simulink model "ClosedLoop_V1"  (R2021b)
settings: Solver=ode4  StartTime=0.0  StopTime=TMax  FixedStep=DT  MaxStep=DT  RelTol=1e-3  EnableMultiTasking=on
undefined symbols (not defined in the file or in its folder): CertificationSettings, Control, DiscIntNeverNeededParam, Drivetrain, OutList, P_InitAngle, RPM_Init, sigbuilder_block, SimConfig, strmatch
libraries: simulink_extras x4, simulink x1
(part 1 of 3)
settings Model: Creator=bjonkman  LastModifiedBy=LaborAdmin
settings SolverCC: AlgebraicLoopSolver=TrustRegion
settings DataIOCC: LimitDataPoints=on  SaveFormat=Array  SignalLoggingSaveFormat=ModelDataLogs  SaveOutput=off  SaveTime=off  ReturnWorkspaceOutputs=off  SignalLoggingName=sigsOut
settings OptimizationCC: ExpressionDepthLimit=2147483647  LifeSpan=inf
settings DebuggingCC: SaveWithParameterizedLinksMsg=none  UnderspecifiedInitializationDetection=Classic  MergeDetectMultiDrivingBlocksExec=none  SignalResolutionControl=TryResolveAllWithWarning  MultiTaskDSMMsg=warning  MultiTaskCondExecSysMsg=none  FcnCallInpInsideContextMsg=warning  StateNameClashWarn=warning  SFUnexpectedBacktrackingDiag=warning  SFNoUnconditionalDefaultTransitionDiag=warning  SFExecutionAtInitializationDiag=none  SFMachineParentedDataDiag=warning  ArithmeticOperatorsInVariantConditions=warning
settings HardwareCC: ProdBitPerPointer=32  ProdBitPerSizeT=32  ProdBitPerPtrDiffT=32  ProdLargestAtomicFloat=None  ProdIntDivRoundTo=Undefined  ProdEndianess=Unspecified  ProdWordSize=32  ProdHWDeviceType=32-bit Generic  TargetUnknown=on
settings ModelReferenceCC: PropagateSignalLabelsOutOfModel=off
settings SFSimCC: SimUseLocalCustomCode=off  CustomCodeUndefinedFunction=UseInterfaceOnly
settings RTWCC: RTWUseLocalCustomCode=off
settings CodeAppCC: StateflowObjectComments=on
settings GRTTargetCC: TargetLangStandard=C89/C90 (ANSI)  CombineOutputUpdateFcns=off  GRTInterface=on
settings ConfigComp: CovMetricSettings=dw  CovSaveCumulativeToWorkspaceVar=on  CovSaveSingleToWorkspaceVar=on  CovExternalEMLEnable=off

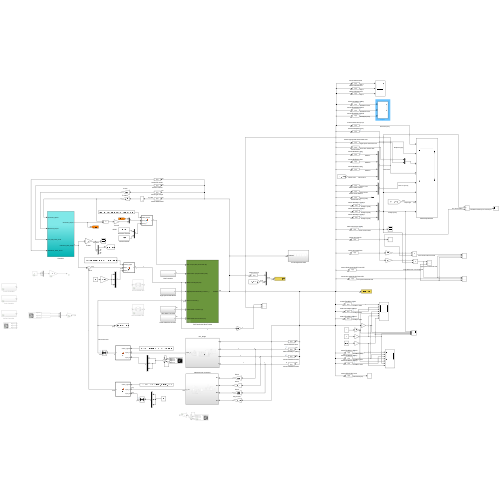
[thumbnail: Simulink's stored preview of the top-level diagram]
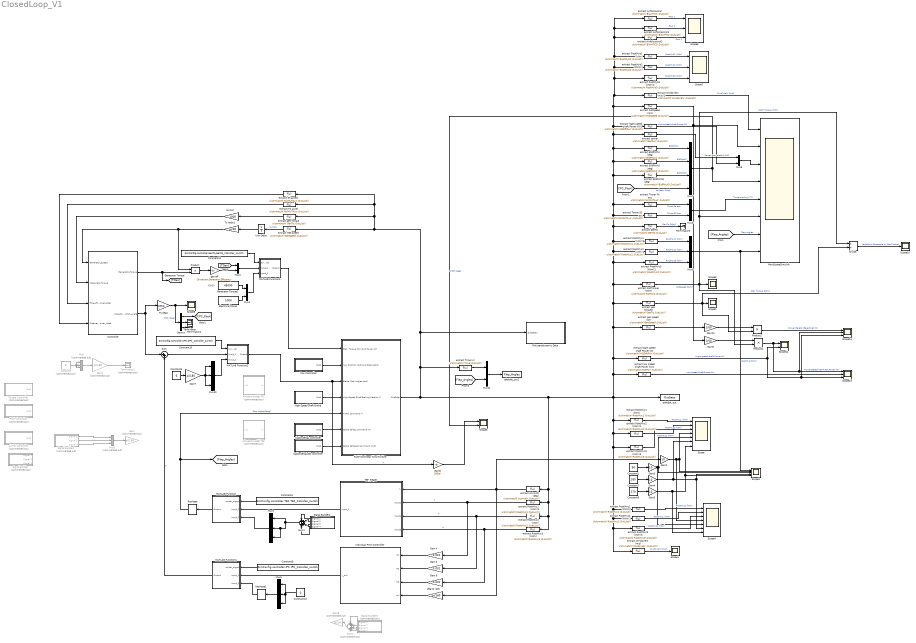
== system ClosedLoop_V1 ==
  note: 43000
  AirFoil Controller : Subsystem  Commented=on
  Aktuatormodell IPC : Subsystem  Commented=on
  Aktuatormodell TEF : Subsystem  Commented=on
  Cable deltaL controller : Subsystem
  Cable deltaLdot controller : Subsystem
  Constant : Constant  Commented=on  Value=6
  Constant1 : Constant  Value=90
  Constant10 : Constant  Value=SimConfig.controller.CPC.CPC_Cotroller_switch
  Constant11 : Constant  Value=SimConfig.controller.GenTq.GenTq_Cotroller_switch
  Constant13 : Constant  Value=0
  Constant3 : Constant  Value=SimConfig.controller.TEF.TEF_Cotroller_switch
  Constant5 : Constant  Value=SimConfig.controller.IPC.IPC_Cotroller_switch
  Constant6 : Constant  Value=6
  Constant7 : Constant  Value=180
  Constant9 : Constant  Value=270
  Controller : Subsystem
  Demux : Demux  Outputs=3
  Divide : Product  Inputs=*/
  Electrical Power : Constant  Value=1000
  FAST Nonlinear Wind Turbine : Subsystem  mask(FAST Nonlinear Wind Turbine){}
      mask help: This block contains the FAST S-Function.
      mask init:
      | clear FAST_SFunc
  Gain : Gain  Commented=on  Gain=pi/180
  Gain 4 : Gain  Gain=0.001
  Gain 5 : Gain  Gain=0.001
  Gain 6 : Gain  Gain=0.001
  Gain1 : Gain  Commented=on  Gain=pi/180
  Gain10 : Gain  Gain=1/60
  Gain{2..5} (4 alike) : Gain  Gain=10
  Gain6 : Gain  Gain=180/pi
  Gain7 : Gain  Gain=pi/180
  Gain8 : Gain  Commented=on  Gain=pi/180
  Gain9 : Gain  Gain=1/60
  Generator Torque2 : Constant  Value=45000
  High-Speed Shaft Brake : Subsystem
  Individual Pitch Controller : Subsystem
  MATLAB Function : MATLAB Function  TreatAsAtomicUnit=on
  MATLAB Function1 : MATLAB Function  TreatAsAtomicUnit=on
  MATLAB Function2 : MATLAB Function  TreatAsAtomicUnit=on
  MATLAB Function3 : MATLAB Function  TreatAsAtomicUnit=on
  MainScopeSimulink : Scope  NumInputPorts=8
  Mux : Mux  Commented=on  Inputs=3
  Mux1 : Mux  Commented=on  Inputs=3
  Mux{3,5,9..10} (4 alike) : Mux  Inputs=3
  Mux{2,4,6,8,11} (5 alike) : Mux  Inputs=2
  Mux7 : Mux
  Pitch Controller : Subsystem  Commented=on
  Plot aerodynamic Data : Subsystem
  Product : Product  RndMeth=Zero
  Product1 : Product
  Product2 : Product
  Reshape : Reshape  OutputDimensionality=Row vector (2-D)  OutputDimensions=[1,3]
  Reshape1 : Reshape  OutputDimensionality=Row vector (2-D)  OutputDimensions=[1,3]
  Scope : Scope  NumInputPorts=7
  Scope{1..2,6,8,15} (5 alike) : Scope
  Scope11 : Scope  NumInputPorts=2
  Scope{7,9,13..14} (4 alike) : Scope  NumInputPorts=3
  Scope3 : Scope  NumInputPorts=5
  Scope4 : Scope  NumInputPorts=7
  Scope5 : Scope  NumInputPorts=2
  Signal Builder : Subsystem  Tag=STV Subsys  Commented=on  LoadFcn=sigbuilder_block('load');  StartFcn=sigbuilder_block('start');  StopFcn=sigbuilder_block('stop');  ClipboardFcn=sigbuilder_block('clipboard');  mask(Sigbuilder block){tuvar=[0:10]}
      mask help: Simulink:masks:SigbuilderBlock_MD
      mask init:
      | if ~strcmp(get_param(bdroot(gcbh),'SimulationStatus'),'stopped') tuvar = sigbuilder_block('maskInit'); end
      settings: CopyFcn=sigbuilder_block('copy');  DeleteFcn=sigbuilder_block('delete');  ModelCloseFcn=sigbuilder_block('modelClose');  PreSaveFcn=sigbuilder_block('preSave');  PauseFcn=sigbuilder_block('pause');  ContinueFcn=sigbuilder_block('continue');  NameChangeFcn=sigbuilder_block('namechange');  OpenFcn=sigbuilder_block('open',[1778.25 246.75 675 420.75 ]);  CloseFcn=sigbuilder_block('close');
      mask Display: plot(0, 0, 100, 100,[2, 2, 32, 32, 2], [68, 8, 8, 68, 68],[32, 2], [38, 38], [32, 19, 2],[53, 60, 44], [32, 17, 17, 2],[16, 16, 31, 31]);txt = getActiveGroup(gcbh);text(2, 100, txt,'verticalAlignment', 'top');
  Signal Builder1 : Subsystem  Tag=STV Subsys  Commented=on  LoadFcn=sigbuilder_block('load');  StartFcn=sigbuilder_block('start');  StopFcn=sigbuilder_block('stop');  ClipboardFcn=sigbuilder_block('clipboard');  mask(Sigbuilder block){tuvar=[0:10]}
      mask help: Simulink:masks:SigbuilderBlock_MD
      mask init:
      | if ~strcmp(get_param(bdroot(gcbh),'SimulationStatus'),'stopped') tuvar = sigbuilder_block('maskInit'); end
      settings: CopyFcn=sigbuilder_block('copy');  DeleteFcn=sigbuilder_block('delete');  ModelCloseFcn=sigbuilder_block('modelClose');  PreSaveFcn=sigbuilder_block('preSave');  PauseFcn=sigbuilder_block('pause');  ContinueFcn=sigbuilder_block('continue');  NameChangeFcn=sigbuilder_block('namechange');  OpenFcn=sigbuilder_block('open',[1778.25 246.75 675 420.75 ]);  CloseFcn=sigbuilder_block('close');
      mask Display: plot(0, 0, 100, 100,[2, 2, 32, 32, 2], [68, 8, 8, 68, 68],[32, 2], [38, 38], [32, 19, 2],[53, 60, 44], [32, 17, 17, 2],[16, 16, 31, 31]);txt = getActiveGroup(gcbh);text(2, 100, txt,'verticalAlignment', 'top');
  Signal Builder2 : Subsystem  Tag=STV Subsys  LoadFcn=sigbuilder_block('load');  StartFcn=sigbuilder_block('start');  StopFcn=sigbuilder_block('stop');  ClipboardFcn=sigbuilder_block('clipboard');  mask(Sigbuilder block){tuvar=[0:10]}
      mask help: Simulink:masks:SigbuilderBlock_MD
      mask init:
      | if ~strcmp(get_param(bdroot(gcbh),'SimulationStatus'),'stopped') tuvar = sigbuilder_block('maskInit'); end
      settings: CopyFcn=sigbuilder_block('copy');  DeleteFcn=sigbuilder_block('delete');  ModelCloseFcn=sigbuilder_block('modelClose');  PreSaveFcn=sigbuilder_block('preSave');  PauseFcn=sigbuilder_block('pause');  ContinueFcn=sigbuilder_block('continue');  NameChangeFcn=sigbuilder_block('namechange');  OpenFcn=sigbuilder_block('open',[881.25 420.75 704.25 505.5 ]);  CloseFcn=sigbuilder_block('close');
      mask Display: plot(0, 0, 100, 100,[2, 2, 32, 32, 2], [68, 8, 8, 68, 68],[32, 2], [38, 38], [32, 19, 2],[53, 60, 44], [32, 17, 17, 2],[16, 16, 31, 31]);txt = getActiveGroup(gcbh);text(2, 100, txt,'verticalAlignment', 'top');
  Signal Builder3 : Subsystem  Tag=STV Subsys  Commented=on  LoadFcn=sigbuilder_block('load');  StartFcn=sigbuilder_block('start');  StopFcn=sigbuilder_block('stop');  ClipboardFcn=sigbuilder_block('clipboard');  mask(Sigbuilder block){tuvar=[0:10]}
      mask help: Simulink:masks:SigbuilderBlock_MD
      mask init:
      | if ~strcmp(get_param(bdroot(gcbh),'SimulationStatus'),'stopped') tuvar = sigbuilder_block('maskInit'); end
      settings: CopyFcn=sigbuilder_block('copy');  DeleteFcn=sigbuilder_block('delete');  ModelCloseFcn=sigbuilder_block('modelClose');  PreSaveFcn=sigbuilder_block('preSave');  PauseFcn=sigbuilder_block('pause');  ContinueFcn=sigbuilder_block('continue');  NameChangeFcn=sigbuilder_block('namechange');  OpenFcn=sigbuilder_block('open',[1807.5 173.25 710.25 410.25 ]);  CloseFcn=sigbuilder_block('close');
      mask Display: plot(0, 0, 100, 100,[2, 2, 32, 32, 2], [68, 8, 8, 68, 68],[32, 2], [38, 38], [32, 19, 2],[53, 60, 44], [32, 17, 17, 2],[16, 16, 31, 31]);txt = getActiveGroup(gcbh);text(2, 100, txt,'verticalAlignment', 'top');
  Sum : Sum  Inputs=|++
  Sum1 : Sum  Inputs=++++
  Sum2 : Sum  Commented=on  Inputs=++++
  TEF_Regler : Subsystem
  Terminator : Terminator
  Terminator1 : Terminator  Commented=on
  Terminator2 : Terminator
  Terminator3 : Terminator
  To deg1 : Gain  Gain=180/pi
  To rad/s1 : Gain  Gain=pi/30
  Torque Controller : Subsystem  Commented=on
  Unit Delay : UnitDelay  InitialCondition=RPM_Init*Drivetrain.Gearbox.Ratio  SampleTime=-1  HasFrameUpgradeWarning=on
  Yaw Controller : Subsystem
  deg to rad1 : Gain  Gain=pi/180
  extract Airfoilcontrol : Fcn  Expr=u(strmatch('BlAirFlC1',OutList))
  extract Airfoilcontrol1 : Fcn  Expr=u(strmatch('BlAirFlC2',OutList))
  extract Airfoilcontrol2 : Fcn  Expr=u(strmatch('BlAirFlC3',OutList))
  extract Azimuth (deg) : Fcn  Expr=u(strmatch('Azimuth',OutList))
  extract BldPitch1 (deg) : Fcn  Expr=u(strmatch('BldPitch1',OutList))
  extract BldPitch2 (deg) : Fcn  Expr=u(strmatch('BldPitch2',OutList))
  extract BldPitch3 (deg) : Fcn  Expr=u(strmatch('BldPitch3',OutList))
  extract FA accel : Fcn  Expr=u(strmatch('NcIMUTAxs',OutList))
  extract GenTq : Fcn  Expr=u(strmatch('GenTq',OutList))
  extract HSS speed : Fcn  Expr=u(strmatch('GenSpeed',OutList))
  extract RootMxc1 (kNm)2 : Fcn  Expr=u(strmatch('RootMxc1',OutList))
  extract RootMxc2 (kNm)1 : Fcn  Expr=u(strmatch('RootMxc2',OutList))
  extract RootMxc3 (kNm)3 : Fcn  Expr=u(strmatch('RootMxc3',OutList))
  extract RootMyb1 (kNm) : Fcn  Expr=u(strmatch('RootMyb1',OutList))
  extract RootMyb1 (kNm)2 : Fcn  Expr=u(strmatch('RootMyb3',OutList))
  extract RootMyb2 (kNm)1 : Fcn  Expr=u(strmatch('RootMyb2',OutList))
  extract RootMyc1 (kNm) : Fcn  Expr=u(strmatch('RootMyc1',OutList))
  extract RootMyc1 (kNm)1 : Fcn  Expr=u(strmatch('RootMyc1',OutList))
  extract RootMyc1 (kNm)3 : Fcn  Expr=u(strmatch('RootMyc1',OutList))
  extract RootMyc2 (kNm) : Fcn  Expr=u(strmatch('RootMyc2',OutList))
  extract RootMyc2 (kNm)1 : Fcn  Expr=u(strmatch('RootMyc2',OutList))
  extract RootMyc2 (kNm)2 : Fcn  Expr=u(strmatch('RootMyc2',OutList))
  extract RootMyc3 (kNm) : Fcn  Expr=u(strmatch('RootMyc3',OutList))
  extract RootMyc3 (kNm)1 : Fcn  Expr=u(strmatch('RootMyc3',OutList))
  extract RootMyc3 (kNm)3 : Fcn  Expr=u(strmatch('RootMyc3',OutList))
  extract RotSpeed (rpm) : Fcn  Expr=u(strmatch('RotSpeed',OutList))
  extract RotTorque (kNm) : Fcn  Expr=u(strmatch('RotTorq',OutList))
  extract SS accel1 : Fcn  Expr=u(strmatch('NcIMUTAys',OutList))
  extract Time (s) : Fcn  Expr=u(strmatch('Time',OutList))
  extract Tower FA acc : Fcn  Expr=u(strmatch('NcIMUTAxs',OutList))
  extract Tower SS acc : Fcn  Expr=u(strmatch('NcIMUTAys',OutList))
  extract Wind1VelX (m/s) : Fcn  Expr=u(strmatch('Wind1VelX',OutList))
  extract Wind1VelX (m/s)1 : Fcn  Expr=u(strmatch('Wind1VelX',OutList))
  extract gen speed rpm : Fcn  Expr=u(strmatch('GenSpeed',OutList))
  extract gen torque : Fcn  Expr=u(strmatch('GenTq',OutList))
  extract gen torque2 : Fcn  Expr=u(strmatch('GenTq',OutList))
  extract hight speed shaft Power kW : Fcn  Expr=u(strmatch('HSShftPwr',OutList))
  extract hight speed shaft Power kW1 : Fcn  Expr=u(strmatch('HSShftPwr',OutList))
  extract low speed shaft Power kW1 : Fcn  Expr=u(strmatch('RotPwr',OutList))
  extract power : Fcn  Expr=u(strmatch('GenPwr',OutList))
  gen eff : Gain  Gain=Drivetrain.Generator.Efficiency
  qdotdot_out : ToWorkspace  VariableName=OutData  SampleTime=-1
  qdotdot_out1 : ToWorkspace  VariableName=Flap_Angles  SampleTime=-1
      settings: Save2DSignal=2-D array (concatenate along first dimension)
  to N/m : Gain  Gain=1000
  wires:
  MATLAB Function3/1(Output) -> FAST Nonlinear Wind Turbine/1(Gen. Torque (Nm) and Power (W))
  Yaw Controller/1(Out1) -> FAST Nonlinear Wind Turbine/2(Yaw Position (rad) and Rate (rad/s))
  Mux1/1 -> Gain/1
  High-Speed Shaft Brake/1(Out1) -> FAST Nonlinear Wind Turbine/4(High-Speed Shaft Braking Fraction (-))
  Cable deltaL controller/1(Out1) -> FAST Nonlinear Wind Turbine/6(Cable deltaL command (m))
  Cable deltaLdot controller/1(Out1) -> FAST Nonlinear Wind Turbine/7(Cable deltaLdot command (m/s))
  extract RootMyc1 (kNm)/1 -> Scope/1  "RootMyc1 (kNm)"
  extract Wind1VelX (m/s)/1 -> Scope1/1  "Wind1VelX [m/s]"
  extract Tower FA acc/1 -> Mux6/1  "Tower Fa acc"
  extract BldPitch2 (deg)/1 -> Mux7/2  "BldPitch2"
  extract Wind1VelX (m/s)1/1 -> MainScopeSimulink/1  "Wind1VelX [m/s]"
  extract GenTq/1 -> Terminator3/1  "GenTq [kNm]"
  Mux6/1 -> MainScopeSimulink/5  "Tower acc [m/s^2]"
  extract BldPitch1 (deg)/1 -> Mux7/1  "BldPitch1"
  extract RotSpeed (rpm)/1 -> Gain9/1, MainScopeSimulink/2  "RotSpeed [rpm]"
  extract BldPitch3 (deg)/1 -> Mux7/3  "BldPitch3"
  extract Tower SS acc/1 -> Mux6/2  "Tower SS acc"
  Reshape/1 -> FAST Nonlinear Wind Turbine/5(AirFoil command (-)), [Flap_Angles]  "Flap Angles [deg]"
  Mux9/1 -> Scope3/1, MainScopeSimulink/8  "RootMyc [kNm]"
  extract power/1 -> Mux8/1  "Power Gen elektrik [kW]"
  Mux7/1 -> MainScopeSimulink/4, Scope5/2  "Pitch [deg]"
  Signal Builder1/3(Signal 3) -> Mux1/3
  Signal Builder1/2(Signal 2) -> Mux1/2
  Signal Builder1/1(Signal 1) -> Mux1/1
  Mux2/1 -> MATLAB Function3/2(Input_1)
  extract gen torque/1 -> to N/m/1
  extract SS accel1/1 -> Controller/4(Sidewards_Tower_Accel)
  [TGen] -> Mux2/1
  gen eff/1 -> Mux2/2
  To rad/s1/1 -> Product/1, Controller/1(Generator_Speed)
  to N/m/1 -> Controller/2(Measured_Torque)
  Mux4/1 -> MATLAB Function3/3(Input_2)
  Product/1 -> gen eff/1
  extract HSS speed/1 -> Unit Delay/1  "W_HSS"
  Controller/1(Generator_Torque) -> [TGen], Product/2
  Unit Delay/1 -> To rad/s1/1
  Constant11/1 -> MATLAB Function3/1(switch_signal)
  extract FA accel/1 -> Controller/3(Fore_Aft_Tower_Accel)
  extract Azimuth (deg)/1 -> Gain2/1, deg to rad1/1, TEF_Regler/1(1)
  extract RootMyc3 (kNm)/1 -> TEF_Regler/4(Input3), Gain 6/1  "H"
  deg to rad1/1 -> Individual Pitch Controller/4(Phi)
  Gain 6/1 -> Individual Pitch Controller/3(M3)
  Gain 5/1 -> Individual Pitch Controller/2(M2)
  Gain 4/1 -> Individual Pitch Controller/1(M1)
  Constant3/1 -> MATLAB Function/1(switch_signal)
  MATLAB Function/1(Output) -> Reshape/1
  TEF_Regler/1(Input_1) -> MATLAB Function/2(Input_1)
  Mux3/1 -> MATLAB Function/3(Input_2)
  [Flap_Angles] -> MainScopeSimulink/7  "Flap Angles"
  Mux5/1 -> Reshape1/1
  Individual Pitch Controller/1(y_out) -> MATLAB Function1/2(Input_1)
  Constant13/1 -> Mux5/3, Mux5/1, Mux5/2
  Constant5/1 -> MATLAB Function1/1(switch_signal)
  Reshape1/1 -> MATLAB Function1/3(Input_2)
  Mux10/1 -> MATLAB Function2/3(Input_2)
  MATLAB Function2/1(Output) -> Gain6/1, FAST Nonlinear Wind Turbine/3(Blade Pitch Angles (rad))  "in"
  Sum/1 -> MATLAB Function2/2(Input_1)
  To deg1/1 -> Demux/1, Scope8/1  "Pitch (deg)"
  Demux/1 -> [CPC_Pitch]
  Demux/3 -> Terminator2/1
  Constant6/1 -> Gain7/1
  Demux/2 -> Terminator/1
  Constant10/1 -> MATLAB Function2/1(switch_signal)
  extract Time (s)/1 -> Mux11/1
  Mux11/1 -> qdotdot_out1/1
  [Flap_Angles] -> Mux11/2
  Controller/2(Collective_Pitch_Angle) -> Sum/1, To deg1/1
  Constant/1 -> Mux/1, Mux/3, Mux/2
  Mux/1 -> Gain1/1
  Gain1/1 -> Terminator1/1
  extract RootMyc2 (kNm)2/1 -> Scope/2  "RootMyc2 (kNm)"
  extract RootMyc3 (kNm)3/1 -> Scope/3  "RootMyc3 (kNm)"
  Gain2/1 -> Scope4/4, Scope3/2, Scope/4
  Constant1/1 -> Gain3/1
  Constant7/1 -> Gain4/1
  Constant9/1 -> Gain5/1
  Gain3/1 -> Scope4/5, Scope/5, Scope3/3
  Gain4/1 -> Scope4/6, Scope3/4, Scope/6
  Gain5/1 -> Scope4/7, Scope3/5, Scope/7
  extract RootMxc1 (kNm)2/1 -> Scope4/1  "RootMxc1 (kNm)"
  extract RootMxc2 (kNm)1/1 -> Scope4/2  "RootMxc1 (kNm)"
  extract RootMxc3 (kNm)3/1 -> Scope4/3  "RootMxc1 (kNm)"
  Gain6/1 -> Scope5/1
  MATLAB Function1/1(Output) -> Sum/2  "F"
  extract RootMyc1 (kNm)1/1 -> TEF_Regler/2(Input1), Gain 4/1  "T"
  extract RootMyc2 (kNm)/1 -> TEF_Regler/3(Input2), Gain 5/1  "T"
  extract RootMyc1 (kNm)3/1 -> Mux9/1  "RootMyc1 (kNm)"
  extract RootMyc2 (kNm)1/1 -> Mux9/2  "RootMyc2 (kNm)"
  extract RootMyc3 (kNm)1/1 -> Mux9/3  "RootMyc3 (kNm)"
  Gain7/1 -> Mux10/1, Mux10/3, Mux10/2
  Generator Torque2/1 -> Mux4/1
  Electrical Power/1 -> Mux4/2
  extract gen torque2/1 -> Divide/2, Product2/2, Scope2/1  "Gen Torque [kNm]"
  Sum1/1 -> Mux3/3, Mux3/2, Mux3/1
  Signal Builder2/3(Signal 3) -> Sum1/3
  Signal Builder2/1(Signal 1) -> Sum1/1
  Signal Builder2/2(Signal 2) -> Sum1/2
  Signal Builder2/4(Signal 4) -> Sum1/4
  Signal Builder3/4(Signal 4) -> Sum2/4
  Signal Builder3/2(Signal 2) -> Sum2/2
  Signal Builder3/1(Signal 1) -> Sum2/1
  Signal Builder3/3(Signal 3) -> Sum2/3
  Sum2/1 -> Gain8/1
  [CPC_Pitch] -> Mux7/4  "collectiv Pitch"
  extract Airfoilcontrol/1 -> Scope9/1  "Flap 1"
  extract Airfoilcontrol1/1 -> Scope9/2  "Flap 2"
  extract Airfoilcontrol2/1 -> Scope9/3  "Flap 3"
  extract RotTorque (kNm)/1 -> Product1/2, Divide/1, MainScopeSimulink/6, Scope6/1  "Rotor Torque (kNm)"
  Gain9/1 -> Product1/1
  Product1/1 -> Scope14/2, Scope13/1, Scope11/1  "Power Berechnet = Rot Power kW"
  extract hight speed shaft Power kW/1 -> Scope11/2, Scope13/3, Scope14/3  "Hight speed shaft Power kW"
  extract low speed shaft Power kW1/1 -> Scope13/2  "Low speed shaft Power kW"
  Gain10/1 -> Product2/1
  extract gen speed rpm/1 -> Gain10/1
  Product2/1 -> Scope14/1  "Power Gerator Berechnet kW"
  extract hight speed shaft Power kW1/1 -> Mux8/2  "Hight speed shaft Power kW"
  Mux8/1 -> MainScopeSimulink/3
  Divide/1 -> Scope15/1  "Verhältnis Rotrtorque zu GenTorque"
  extract RootMyb1 (kNm)/1 -> Scope7/1  "RootMyb1 (kNm)"
  extract RootMyb2 (kNm)1/1 -> Scope7/2  "RootMyb2 (kNm)"
  extract RootMyb1 (kNm)2/1 -> Scope7/3  "RootMyb3 (kNm)"
  FAST Nonlinear Wind Turbine/1(OutData) -> extract Time (s)/1, Plot aerodynamic Data/1(OutData1), extract HSS speed/1, extract gen torque/1, extract FA accel/1, extract SS accel1/1, extract RootMyc2 (kNm)/1, extract RootMyc3 (kNm)/1, extract RootMyc1 (kNm)1/1, extract Azimuth (deg)/1, extract RootMyc2 (kNm)2/1, extract RootMyc3 (kNm)3/1, extract RootMxc1 (kNm)2/1, extract RootMxc2 (kNm)1/1, extract RootMxc3 (kNm)3/1, extract Wind1VelX (m/s)/1, extract RootMyc1 (kNm)/1, extract low speed shaft Power kW1/1, extract hight speed shaft Power kW/1, extract gen speed rpm/1, extract gen torque2/1, extract RotTorque (kNm)/1, extract RootMyc3 (kNm)1/1, extract RootMyc2 (kNm)1/1, extract RootMyc1 (kNm)3/1, extract GenTq/1, extract Tower SS acc/1, extract Tower FA acc/1, extract hight speed shaft Power kW1/1, extract RotSpeed (rpm)/1, extract RootMyb1 (kNm)2/1, extract RootMyb2 (kNm)1/1, extract RootMyb1 (kNm)/1, extract Airfoilcontrol2/1, extract Airfoilcontrol1/1, extract Airfoilcontrol/1, extract Wind1VelX (m/s)1/1, extract power/1, extract BldPitch1 (deg)/1, extract BldPitch2 (deg)/1, extract BldPitch3 (deg)/1, qdotdot_out/1

== system ClosedLoop_V1/AirFoil Controller ==
  Airfoil command : Constant  Value=zeros(1,3)'
  Out1 : Outport
  wires:
  Airfoil command/1 -> Out1/1

== system ClosedLoop_V1/Aktuatormodell IPC ==
  In1 : Inport
  Demux2 : Demux  Outputs=3
  Mux13 : Mux  Inputs=3
  Transfer Fcn3 : TransferFcn  Denominator=[0.1 1]
  Transfer Fcn4 : TransferFcn  Denominator=[0.1 1]
  Transfer Fcn5 : TransferFcn  Denominator=[0.1 1]
  in : Outport
  wires:
  In1/1 -> Demux2/1
  Demux2/3 -> Transfer Fcn4/1
  Transfer Fcn3/1 -> Mux13/2  "T"
  Demux2/1 -> Transfer Fcn5/1
  Demux2/2 -> Transfer Fcn3/1
  Transfer Fcn5/1 -> Mux13/1  "T"
  Transfer Fcn4/1 -> Mux13/3  "T"
  Mux13/1 -> in/1  "in"

== system ClosedLoop_V1/Aktuatormodell TEF ==
  In1 : Inport
  Demux2 : Demux  Outputs=3
  Mux13 : Mux  Inputs=3
  Transfer Fcn3 : TransferFcn  Denominator=[0.04 1]
  Transfer Fcn4 : TransferFcn  Denominator=[0.04 1]
  Transfer Fcn5 : TransferFcn  Denominator=[0.04 1]
  in : Outport
  wires:
  Mux13/1 -> in/1  "in"
  Transfer Fcn4/1 -> Mux13/3  "T"
  Transfer Fcn5/1 -> Mux13/1  "T"
  Demux2/2 -> Transfer Fcn3/1
  Demux2/1 -> Transfer Fcn5/1
  Transfer Fcn3/1 -> Mux13/2  "T"
  Demux2/3 -> Transfer Fcn4/1
  In1/1 -> Demux2/1

== system ClosedLoop_V1/Cable deltaL controller ==
  Cable deltaL command : Constant  Value=zeros(1,20)'
  Out1 : Outport
  wires:
  Cable deltaL command/1 -> Out1/1

== system ClosedLoop_V1/Cable deltaLdot controller ==
  Cable deltaLdot command : Constant  Value=zeros(1,20)'
  Out1 : Outport
  wires:
  Cable deltaLdot command/1 -> Out1/1

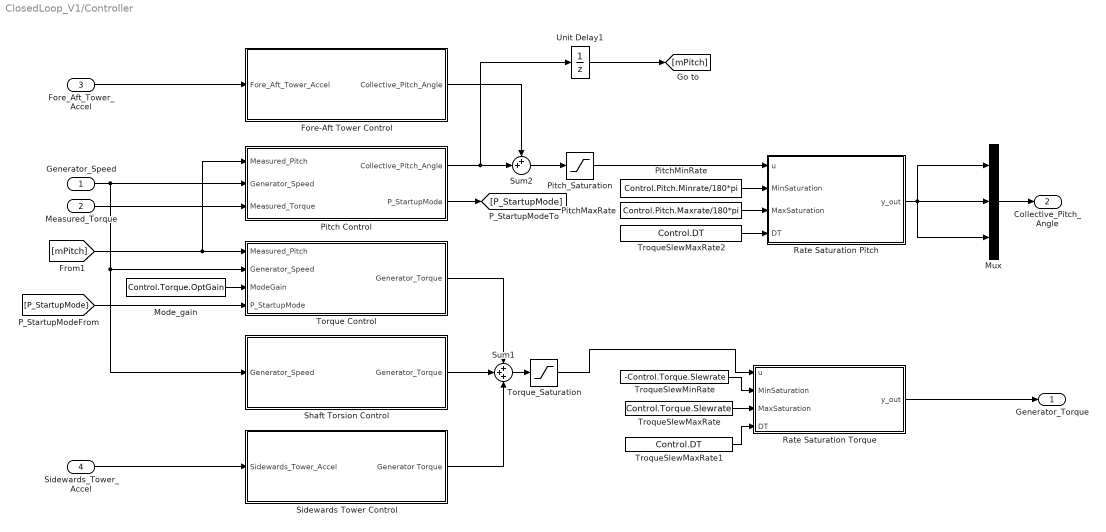
== system ClosedLoop_V1/Controller ==
  Generator_Speed : Inport
  Measured_Torque : Inport  Port=2
  Fore_Aft_Tower_Accel : Inport  Port=3
  Sidewards_Tower_Accel : Inport  Port=4  PortDimensions=1
  Fore-Aft Tower Control : Subsystem
  Mode_gain : Constant  Value=Control.Torque.OptGain
  Mux : Mux  Inputs=3
  Pitch Control : Subsystem
  PitchMaxRate : Constant  Value=Control.Pitch.Maxrate/180*pi
  PitchMinRate : Constant  Value=Control.Pitch.Minrate/180*pi
  Pitch_Saturation : Saturate  UpperLimit=Control.Pitch.Max*pi/180  LowerLimit=Control.Pitch.Min*pi/180
  Rate Saturation Pitch : MATLAB Function  TreatAsAtomicUnit=on
  Rate Saturation Torque : MATLAB Function  TreatAsAtomicUnit=on
  Shaft Torsion Control : Subsystem
  Sidewards Tower Control : Subsystem
  Sum1 : Sum  Inputs=+++
  Sum2 : Sum  Inputs=++|
  Torque Control : Subsystem
  Torque_Saturation : Saturate  UpperLimit=Control.Torque.Limit  LowerLimit=Control.Torque.Min
  TroqueSlewMaxRate : Constant  Value=Control.Torque.Slewrate
  TroqueSlewMaxRate1 : Constant  Value=Control.DT
  TroqueSlewMaxRate2 : Constant  Value=Control.DT
  TroqueSlewMinRate : Constant  Value=-Control.Torque.Slewrate
  Unit Delay1 : UnitDelay  InitialCondition=P_InitAngle*pi/180  SampleTime=-1  HasFrameUpgradeWarning=on
  Generator_Torque : Outport  VectorParamsAs1DForOutWhenUnconnected=off
  Collective_Pitch_Angle : Outport  Port=2  PortDimensions=3  VectorParamsAs1DForOutWhenUnconnected=off
  wires:
  Sidewards_Tower_Accel/1 -> Sidewards Tower Control/1(Sidewards_Tower_Accel)
  Fore_Aft_Tower_Accel/1 -> Fore-Aft Tower Control/1(Fore_Aft_Tower_Accel)
  Fore-Aft Tower Control/1(Collective_Pitch_Angle) -> Sum2/1
  Torque Control/1(Generator_Torque) -> Sum1/1
  Sidewards Tower Control/1(Generator Torque) -> Sum1/3
  [mPitch] -> Pitch Control/1(Measured_Pitch), Torque Control/1(Measured_Pitch)
  Measured_Torque/1 -> Pitch Control/3(Measured_Torque)
  Shaft Torsion Control/1(Generator_Torque) -> Sum1/2
  Mode_gain/1 -> Torque Control/3(ModeGain)
  Sum1/1 -> Torque_Saturation/1
  Mux/1 -> Collective_Pitch_Angle/1
  Unit Delay1/1 -> [mPitch]
  Sum2/1 -> Pitch_Saturation/1
  Rate Saturation Pitch/1(y_out) -> Mux/3, Mux/2, Mux/1
  PitchMinRate/1 -> Rate Saturation Pitch/2(MinSaturation)
  PitchMaxRate/1 -> Rate Saturation Pitch/3(MaxSaturation)
  Pitch_Saturation/1 -> Rate Saturation Pitch/1(u)
  TroqueSlewMinRate/1 -> Rate Saturation Torque/2(MinSaturation)
  TroqueSlewMaxRate/1 -> Rate Saturation Torque/3(MaxSaturation)
  Generator_Speed/1 -> Pitch Control/2(Generator_Speed), Torque Control/2(Generator_Speed), Shaft Torsion Control/1(Generator_Speed)
  [P_StartupMode] -> Torque Control/4(P_StartupMode)
  Pitch Control/2(P_StartupMode) -> [P_StartupMode]
  Pitch Control/1(Collective_Pitch_Angle) -> Sum2/2, Unit Delay1/1
  TroqueSlewMaxRate1/1 -> Rate Saturation Torque/4(DT)
  TroqueSlewMaxRate2/1 -> Rate Saturation Pitch/4(DT)
  Torque_Saturation/1 -> Rate Saturation Torque/1(u)
  Rate Saturation Torque/1(y_out) -> Generator_Torque/1

== system ClosedLoop_V1/FAST Nonlinear Wind Turbine ==
  Gen. Torque (Nm) and Power (W) : Inport
  Yaw Position (rad) and Rate (rad/s) : Inport  Port=2
  Blade Pitch Angles (rad) : Inport  Port=3
  High-Speed Shaft Braking Fraction (-) : Inport  Port=4
  AirFoil command (-) : Inport  Port=5
  Cable deltaL command (m) : Inport  Port=6
  Cable deltaLdot command (m/s) : Inport  Port=7
  Mux1 : Mux  Inputs=7
  S-Function : S-Function  FunctionName=FAST_SFunc  Parameters=FAST_InputFileName, TMax, 0  SFunctionDeploymentMode=off  EnableBusSupport=off
  Signal Specification1 : SignalSpecification  OutDataTypeStr=double  Dimensions=2
  Signal Specification2 : SignalSpecification  OutDataTypeStr=double  Dimensions=2
  OutData : Outport
  wires:
  Gen. Torque (Nm) and Power (W)/1 -> Signal Specification1/1
  S-Function/1 -> OutData/1
  Mux1/1 -> S-Function/1
  Blade Pitch Angles (rad)/1 -> Mux1/3
  Yaw Position (rad) and Rate (rad/s)/1 -> Signal Specification2/1
  Signal Specification1/1 -> Mux1/1
  Signal Specification2/1 -> Mux1/2
  High-Speed Shaft Braking Fraction (-)/1 -> Mux1/4
  AirFoil command (-)/1 -> Mux1/5
  Cable deltaL command (m)/1 -> Mux1/6
  Cable deltaLdot command (m/s)/1 -> Mux1/7

== system ClosedLoop_V1/High-Speed Shaft Brake ==
  High-Speed Shaft Braking Fraction : Constant  Value=0
  Out1 : Outport
  wires:
  High-Speed Shaft Braking Fraction/1 -> Out1/1

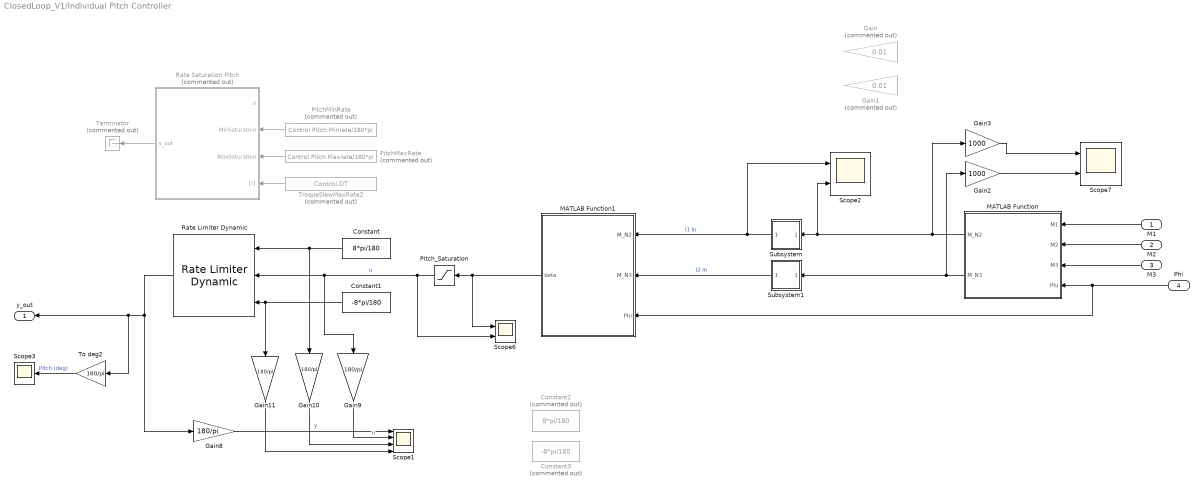
== system ClosedLoop_V1/Individual Pitch Controller ==
  M1 : Inport
  M2 : Inport  Port=2
  M3 : Inport  Port=3
  Phi : Inport  Port=4
  Constant : Constant  Value=8*pi/180
  Constant1 : Constant  Value=-8*pi/180
  Constant2 : Constant  Commented=on  Value=8*pi/180
  Constant3 : Constant  Commented=on  Value=-8*pi/180
  Gain : Gain  Commented=on  Gain=0.01
  Gain1 : Gain  Commented=on  Gain=0.01
  Gain{8..11} (4 alike) : Gain  Gain=180/pi
  Gain2 : Gain  Gain=1000
  Gain3 : Gain  Gain=1000
  MATLAB Function : MATLAB Function  TreatAsAtomicUnit=on
  MATLAB Function1 : MATLAB Function  TreatAsAtomicUnit=on
  PitchMaxRate : Constant  Commented=on  Value=Control.Pitch.Maxrate/180*pi
  PitchMinRate : Constant  Commented=on  Value=Control.Pitch.Minrate/180*pi
  Pitch_Saturation : Saturate  UpperLimit=Control.Pitch.Max*pi/180  LowerLimit=Control.Pitch.Min*pi/180
  Rate Limiter Dynamic : simulink/Discontinuities/Rate Limiter Dynamic
  Rate Saturation Pitch : MATLAB Function  Commented=on  TreatAsAtomicUnit=on
  Scope1 : Scope  NumInputPorts=4
  Scope2 : Scope  NumInputPorts=2
  Scope3 : Scope
  Scope6 : Scope  NumInputPorts=2
  Scope7 : Scope  NumInputPorts=2
  Subsystem : Subsystem
  Subsystem1 : Subsystem
  Terminator : Terminator  Commented=on
  To deg2 : Gain  Gain=180/pi
  TroqueSlewMaxRate2 : Constant  Commented=on  Value=Control.DT
  y_out : Outport
  wires:
  MATLAB Function1/1(beta) -> Pitch_Saturation/1, Scope6/1
  M1/1 -> MATLAB Function/1(M1)
  M2/1 -> MATLAB Function/2(M2)
  To deg2/1 -> Scope3/1  "Pitch (deg)"
  MATLAB Function/1(M_N2) -> Scope2/2, Subsystem/1(M_N2), Gain3/1
  Gain2/1 -> Scope7/2
  M3/1 -> MATLAB Function/3(M3)
  TroqueSlewMaxRate2/1 -> Rate Saturation Pitch/4(DT)
  Rate Limiter Dynamic/1 -> Gain8/1, To deg2/1, y_out/1
  Pitch_Saturation/1 -> Scope6/2, Rate Limiter Dynamic/2, Gain9/1  "u"
  MATLAB Function/2(M_N3) -> Subsystem1/1(M_N3), Gain2/1
  PitchMaxRate/1 -> Rate Saturation Pitch/3(MaxSaturation)
  Phi/1 -> MATLAB Function1/3(Phi), MATLAB Function/4(Phi)
  PitchMinRate/1 -> Rate Saturation Pitch/2(MinSaturation)
  Gain3/1 -> Scope7/1
  Subsystem/1(Out1) -> Scope2/1, MATLAB Function1/1(M_N2)  "I1 in"
  Subsystem1/1(Out1) -> MATLAB Function1/2(M_N3)  "I2 in"
  Gain11/1 -> Scope1/4
  Gain10/1 -> Scope1/3
  Gain9/1 -> Scope1/2  "u"
  Gain8/1 -> Scope1/1  "y"
  Constant/1 -> Rate Limiter Dynamic/1, Gain10/1
  Constant1/1 -> Gain11/1, Rate Limiter Dynamic/3
  Rate Saturation Pitch/1(y_out) -> Terminator/1

== system ClosedLoop_V1/Pitch Controller ==
  Blade Pitch Angles : Constant  Commented=on  Value=zeros(1,3)'
  Constant : Constant  Value=8
  Gain : Gain  Gain=pi/180
  Mux : Mux  Inputs=3
  Out1 : Outport
  wires:
  Constant/1 -> Mux/2, Mux/3, Mux/1
  Mux/1 -> Gain/1
  Gain/1 -> Out1/1

== system ClosedLoop_V1/Plot aerodynamic Data ==
  OutData1 : Inport
  Plot Angle of Attack : Subsystem
  Plot Cd : Subsystem
  Plot Cl : Subsystem
  Plot Pitch+Twist Angle : Subsystem
  Plot Reynolds number : Subsystem
  Plot Rotor Data : Subsystem
  wires:
  OutData1/1 -> Plot Reynolds number/1(OutData1), Plot Angle of Attack/1(OutData), Plot Pitch+Twist Angle/1(OutData), Plot Cl/2(OutData1), Plot Cl/1(OutData), Plot Cd/1(OutData), Plot Rotor Data/1(OutData)

== system ClosedLoop_V1/Signal Builder ==
  Demux : Demux  Tag=STV Demux  Outputs=3
      settings: DisplayOption=none
  FromWs : FromWorkspace  Tag=STV FromWs  VariableName=tuvar
      SigBuilderData=|
      | common.afterFinalStr = 'Extrapolate'
      | common.sampleTime = 0
      | dataSet.timeRange = [0 60]
      | dataSet.name = 'Group 1'
      | sbobj.Groups.Name = 'Group 1'
      | sbobj.Groups.Signals(1).Name = 'Signal 1'
      | sbobj.Groups.Signals(1).XData = [0 15.7 15.7 23.3 23.3 60]
      | sbobj.Groups.Signals(1).YData = [0 0 10 10 0 0]
      | sbobj.Groups.Signals(2).Name = 'Signal 2'
      | sbobj.Groups.Signals(2).XData = [0 29.4 29.4 36 36 60]
      | sbobj.Groups.Signals(2).YData = [0 0 1 1 0 0]
      | sbobj.Groups.Signals(3).Name = 'Signal 3'
      | sbobj.Groups.Signals(3).XData = [0 43.4 43.4 50.8 50.8 60]
      | sbobj.Groups.Signals(3).YData = [0 0 -5.1 -5.1 0 0]
      | sbobj.Groups.TimeRange = [0 60]
  Signal 1 : Outport  Tag=STV Outport
  Signal 2 : Outport  Tag=STV Outport  Port=2
  Signal 3 : Outport  Tag=STV Outport  Port=3
  wires:
  Demux/1 -> Signal 1/1
  FromWs/1 -> Demux/1
  Demux/2 -> Signal 2/1
  Demux/3 -> Signal 3/1

== system ClosedLoop_V1/Signal Builder1 ==
  Demux : Demux  Tag=STV Demux  Outputs=3
      settings: DisplayOption=none
  FromWs : FromWorkspace  Tag=STV FromWs  VariableName=tuvar
      SigBuilderData=|
      | common.afterFinalStr = 'Extrapolate'
      | common.sampleTime = 0
      | dataSet.timeRange = [0 60]
      | dataSet.name = 'Group 1'
      | sbobj.Groups.Name = 'Group 1'
      | sbobj.Groups.Signals(1).Name = 'Signal 1'
      | sbobj.Groups.Signals(1).XData = [0 15.7 15.7 23.3 23.3 60]
      | sbobj.Groups.Signals(1).YData = [0 0 10 10 0 0]
      | sbobj.Groups.Signals(2).Name = 'Signal 2'
      | sbobj.Groups.Signals(2).XData = [0 29.4 29.4 36 36 60]
      | sbobj.Groups.Signals(2).YData = [0 0 1 1 0 0]
      | sbobj.Groups.Signals(3).Name = 'Signal 3'
      | sbobj.Groups.Signals(3).XData = [0 43.4 43.4 50.8 50.8 60]
      | sbobj.Groups.Signals(3).YData = [0 0 -5.1 -5.1 0 0]
      | sbobj.Groups.TimeRange = [0 60]
  Signal 1 : Outport  Tag=STV Outport
  Signal 2 : Outport  Tag=STV Outport  Port=2
  Signal 3 : Outport  Tag=STV Outport  Port=3
  wires:
  Demux/3 -> Signal 3/1
  Demux/2 -> Signal 2/1
  FromWs/1 -> Demux/1
  Demux/1 -> Signal 1/1

== system ClosedLoop_V1/Signal Builder2 ==
  Demux : Demux  Tag=STV Demux
      settings: DisplayOption=none
  FromWs : FromWorkspace  Tag=STV FromWs  VariableName=tuvar
      SigBuilderData=|
      | common.afterFinalStr = 'Extrapolate'
      | common.sampleTime = 0
      | dataSet.timeRange = [0 600]
      | dataSet.name = 'Group 1'
      | sbobj.Groups.Name = 'Group 1'
      | sbobj.Groups.Signals(1).Name = 'Signal 1'
      | sbobj.Groups.Signals(1).XData = [0 100 100 150 150 600]
      | sbobj.Groups.Signals(1).YData = [0 0 2 2 0 0]
      | sbobj.Groups.Signals(2).Name = 'Signal 2'
      | sbobj.Groups.Signals(2).XData = [0 200 200 250 250 600]
      | sbobj.Groups.Signals(2).YData = [0 0 -2 -2 0 0]
      | sbobj.Groups.Signals(3).Name = 'Signal 3'
      | sbobj.Groups.Signals(3).XData = [0 300 300 350 350 600]
      | sbobj.Groups.Signals(3).YData = [0 0 5 5 0 0]
      | sbobj.Groups.Signals(4).Name = 'Signal 4'
      | sbobj.Groups.Signals(4).XData = [0 400 400 450 450 600]
      | sbobj.Groups.Signals(4).YData = [0 0 -5 -5 0 0]
      | sbobj.Groups.TimeRange = [0 600]
  Signal 1 : Outport  Tag=STV Outport
  Signal 2 : Outport  Tag=STV Outport  Port=2
  Signal 3 : Outport  Tag=STV Outport  Port=3
  Signal 4 : Outport  Tag=STV Outport  Port=4
  wires:
  Demux/1 -> Signal 1/1
  FromWs/1 -> Demux/1
  Demux/2 -> Signal 2/1
  Demux/3 -> Signal 3/1
  Demux/4 -> Signal 4/1

== system ClosedLoop_V1/Signal Builder3 ==
  Demux : Demux  Tag=STV Demux
      settings: DisplayOption=none
  FromWs : FromWorkspace  Tag=STV FromWs  VariableName=tuvar
      SigBuilderData=|
      | common.afterFinalStr = 'Extrapolate'
      | common.sampleTime = 0
      | dataSet.timeRange = [0 600]
      | dataSet.name = 'Group 1'
      | sbobj.Groups.Name = 'Group 1'
      | sbobj.Groups.Signals(1).Name = 'Signal 1'
      | sbobj.Groups.Signals(1).XData = [0 100 100 150 150 600]
      | sbobj.Groups.Signals(1).YData = [0 0 4 4 0 0]
      | sbobj.Groups.Signals(2).Name = 'Signal 2'
      | sbobj.Groups.Signals(2).XData = [0 200 200 250 250 600]
      | sbobj.Groups.Signals(2).YData = [0 0 -4 -4 0 0]
      | sbobj.Groups.Signals(3).Name = 'Signal 3'
      | sbobj.Groups.Signals(3).XData = [0 300 300 350 350 600]
      | sbobj.Groups.Signals(3).YData = [0 0 2 2 0 0]
      | sbobj.Groups.Signals(4).Name = 'Signal 4'
      | sbobj.Groups.Signals(4).XData = [0 400 400 450 450 600]
      | sbobj.Groups.Signals(4).YData = [0 0 -2 -2 0 0]
      | sbobj.Groups.TimeRange = [0 600]
  Signal 1 : Outport  Tag=STV Outport
  Signal 2 : Outport  Tag=STV Outport  Port=2
  Signal 3 : Outport  Tag=STV Outport  Port=3
  Signal 4 : Outport  Tag=STV Outport  Port=4
  wires:
  Demux/1 -> Signal 1/1
  FromWs/1 -> Demux/1
  Demux/2 -> Signal 2/1
  Demux/3 -> Signal 3/1
  Demux/4 -> Signal 4/1

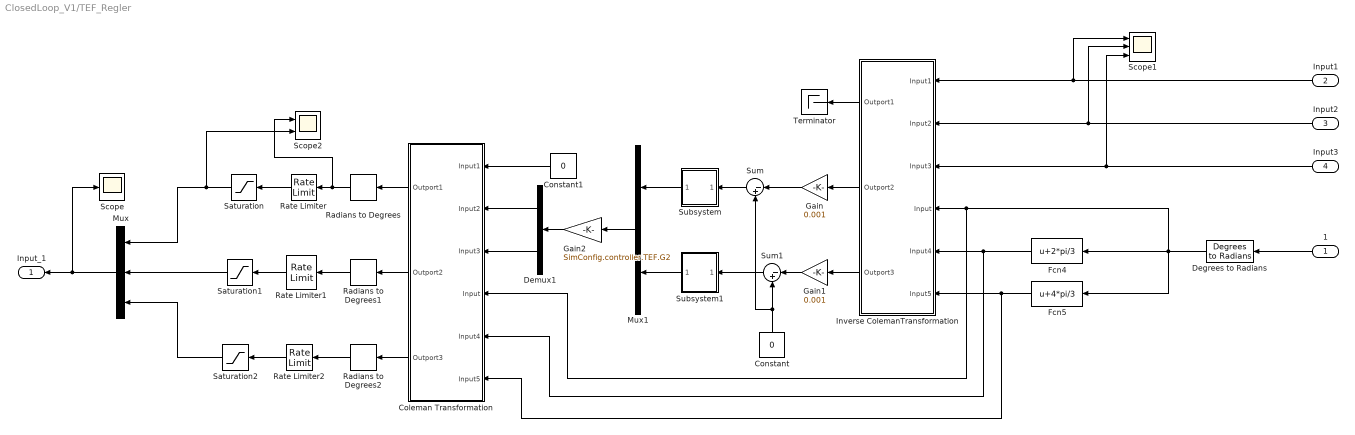
== system ClosedLoop_V1/TEF_Regler ==
  1 : Inport
  Input1 : Inport  Port=2
  Input2 : Inport  Port=3
  Input3 : Inport  Port=4
  Coleman Transformation : Subsystem
  Constant : Constant  Value=0
  Constant1 : Constant  Value=0
  Degrees to Radians : simulink_extras/Transformations/Degrees to Radians
  Demux1 : Demux  Outputs=2
  Fcn4 : Fcn  Expr=u+2*pi/3
  Fcn5 : Fcn  Expr=u+4*pi/3
  Gain : Gain  Gain=0.001
  Gain1 : Gain  Gain=0.001
  Gain2 : Gain  Gain=SimConfig.controller.TEF.G2
  Inverse ColemanTransformation : Subsystem
  Mux : Mux  Inputs=3
  Mux1 : Mux  Inputs=2
  Radians to Degrees : simulink_extras/Transformations/Radians to Degrees
  Radians to Degrees1 : simulink_extras/Transformations/Radians to Degrees
  Radians to Degrees2 : simulink_extras/Transformations/Radians to Degrees
  Rate Limiter : RateLimiter  RisingSlewLimit=20  FallingSlewLimit=-20  SampleTimeMode=inherited
  Rate Limiter1 : RateLimiter  RisingSlewLimit=20  FallingSlewLimit=-20  SampleTimeMode=inherited
  Rate Limiter2 : RateLimiter  RisingSlewLimit=20  FallingSlewLimit=-20  SampleTimeMode=inherited
  Saturation : Saturate  UpperLimit=10  LowerLimit=-10
  Saturation1 : Saturate  UpperLimit=10  LowerLimit=-10
  Saturation2 : Saturate  UpperLimit=10  LowerLimit=-10
  Scope : Scope
  Scope1 : Scope  NumInputPorts=3
  Scope2 : Scope  NumInputPorts=2
  Subsystem : Subsystem
  Subsystem1 : Subsystem
  Sum : Sum  Inputs=|-+
  Sum1 : Sum  Inputs=|-+
  Terminator : Terminator
  Input_1 : Outport
  wires:
  Coleman Transformation/3(Outport3) -> Radians to Degrees2/1
  1/1 -> Degrees to Radians/1
  Constant/1 -> Sum/2, Sum1/2
  Degrees to Radians/1 -> Coleman Transformation/4(Input), Inverse ColemanTransformation/4(Input), Fcn4/1, Fcn5/1
  Inverse ColemanTransformation/1(Outport1) -> Terminator/1
  Subsystem1/1(Out1) -> Mux1/2
  Rate Limiter1/1 -> Saturation1/1
  Fcn5/1 -> Coleman Transformation/6(Input5), Inverse ColemanTransformation/6(Input5)
  Coleman Transformation/2(Outport2) -> Radians to Degrees1/1
  Saturation/1 -> Scope2/2, Mux/1
  Fcn4/1 -> Coleman Transformation/5(Input4), Inverse ColemanTransformation/5(Input4)
  Gain2/1 -> Demux1/1
  Inverse ColemanTransformation/2(Outport2) -> Gain/1
  Radians to Degrees1/1 -> Rate Limiter1/1
  Radians to Degrees2/1 -> Rate Limiter2/1
  Sum1/1 -> Subsystem1/1(In1)
  Rate Limiter2/1 -> Saturation2/1
  Inverse ColemanTransformation/3(Outport3) -> Gain1/1
  Saturation1/1 -> Mux/2
  Rate Limiter/1 -> Saturation/1
  Radians to Degrees/1 -> Scope2/1, Rate Limiter/1
  Saturation2/1 -> Mux/3
  Gain1/1 -> Sum1/1
  Gain/1 -> Sum/1
  Sum/1 -> Subsystem/1(In1)
  Mux1/1 -> Gain2/1
  Demux1/1 -> Coleman Transformation/2(Input2)
  Constant1/1 -> Coleman Transformation/1(Input1)
  Subsystem/1(Out1) -> Mux1/1
  Demux1/2 -> Coleman Transformation/3(Input3)
  Coleman Transformation/1(Outport1) -> Radians to Degrees/1
  Input1/1 -> Scope1/1, Inverse ColemanTransformation/1(Input1)
  Input2/1 -> Scope1/2, Inverse ColemanTransformation/2(Input2)
  Mux/1 -> Scope/1, Input_1/1
  Input3/1 -> Inverse ColemanTransformation/3(Input3), Scope1/3

== system ClosedLoop_V1/Torque Controller ==
  Electrical Power : Constant  Value=5000000
  Generator Torque : Constant  Value=1000
  Mux : Mux  Inputs=2
  Out1 : Outport
  wires:
  Mux/1 -> Out1/1
  Generator Torque/1 -> Mux/1
  Electrical Power/1 -> Mux/2

== system ClosedLoop_V1/Yaw Controller ==
  Mux : Mux  Inputs=2
  Yaw Position : Constant  Value=0
  Yaw rate : Constant  Value=0
  Out1 : Outport
  wires:
  Mux/1 -> Out1/1
  Yaw Position/1 -> Mux/1
  Yaw rate/1 -> Mux/2

== system ClosedLoop_V1/Controller/Fore-Aft Tower Control ==
  note: Fore-Aft tower damping
  Fore_Aft_Tower_Accel : Inport
  Discrete-Time Integrator : DiscreteIntegrator  SampleTime=-1  ICPrevOutput=DiscIntNeverNeededParam  ICPrevScaledInput=DiscIntNeverNeededParam
  Gain1 : Gain  Gain=Control.ForeAft.Gain
  Pitch_Saturation : Saturate  UpperLimit=Control.ForeAft.MaxPitchAmplitude*pi/180  LowerLimit=-Control.ForeAft.MaxPitchAmplitude*pi/180
  Scope : Scope  NumInputPorts=2
  Scope1 : Scope  NumInputPorts=2
  Collective_Pitch_Angle : Outport  VectorParamsAs1DForOutWhenUnconnected=off
  wires:
  Fore_Aft_Tower_Accel/1 -> Scope/2, Discrete-Time Integrator/1  "in"
  Pitch_Saturation/1 -> Scope1/2, Collective_Pitch_Angle/1
  Discrete-Time Integrator/1 -> Gain1/1, Scope/1  "out"
  Gain1/1 -> Pitch_Saturation/1, Scope1/1

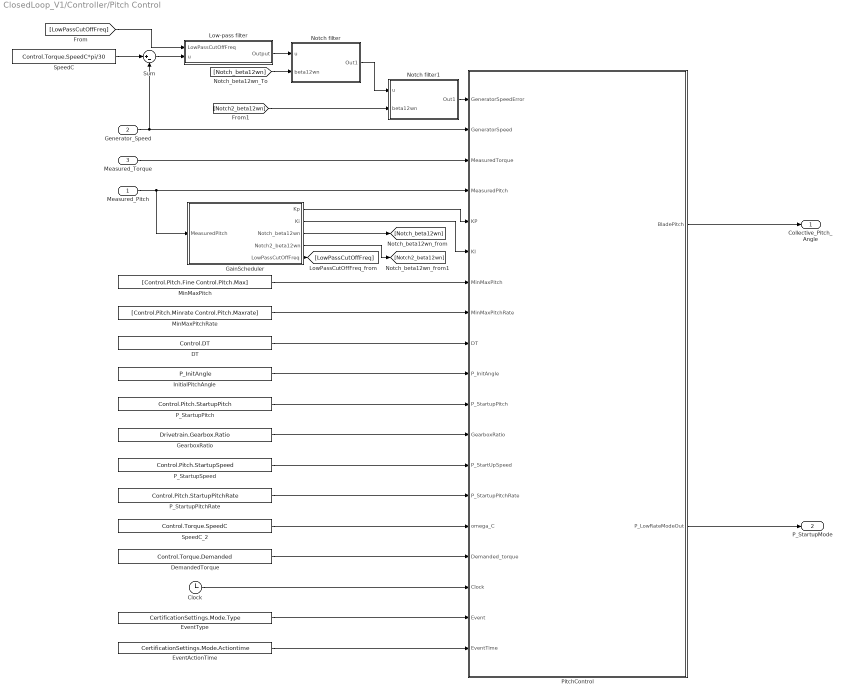
== system ClosedLoop_V1/Controller/Pitch Control ==
  Measured_Pitch : Inport
  Generator_Speed : Inport  Port=2
  Measured_Torque : Inport  Port=3
  Clock : Clock
  DT : Constant  Value=Control.DT
  DemandedTorque : Constant  Value=Control.Torque.Demanded
  EventActionTime : Constant  Value=CertificationSettings.Mode.Actiontime
  EventType : Constant  Value=CertificationSettings.Mode.Type
  GainScheduler : Subsystem
  GearboxRatio : Constant  Value=Drivetrain.Gearbox.Ratio
  InitialPitchAngle : Constant  Value=P_InitAngle
  Low-pass filter : Subsystem
  MinMaxPitch : Constant  Value=[Control.Pitch.Fine Control.Pitch.Max]
  MinMaxPitchRate : Constant  Value=[Control.Pitch.Minrate Control.Pitch.Maxrate]
  Notch filter : Subsystem
  Notch filter1 : Subsystem
  P_StartupPitch : Constant  Value=Control.Pitch.StartupPitch
  P_StartupPitchRate : Constant  Value=Control.Pitch.StartupPitchRate
  P_StartupSpeed : Constant  Value=Control.Pitch.StartupSpeed
  PitchControl : MATLAB Function  TreatAsAtomicUnit=on
  SpeedC : Constant  Value=Control.Torque.SpeedC*pi/30
  SpeedC_2 : Constant  Value=Control.Torque.SpeedC
  Sum : Sum  Inputs=|+-
  Collective_Pitch_Angle : Outport  VectorParamsAs1DForOutWhenUnconnected=off
  P_StartupMode : Outport  Port=2  VectorParamsAs1DForOutWhenUnconnected=off
  wires:
  MinMaxPitch/1 -> PitchControl/7(MinMaxPitch)
  MinMaxPitchRate/1 -> PitchControl/8(MinMaxPitchRate)
  PitchControl/1(BladePitch) -> Collective_Pitch_Angle/1
  Measured_Torque/1 -> PitchControl/3(MeasuredTorque)
  SpeedC/1 -> Sum/1
  Generator_Speed/1 -> PitchControl/2(GeneratorSpeed), Sum/2
  Sum/1 -> Low-pass filter/2(u)
  PitchControl/2(P_LowRateModeOut) -> P_StartupMode/1
  DT/1 -> PitchControl/9(DT)
  P_StartupPitch/1 -> PitchControl/11(P_StartupPitch)
  InitialPitchAngle/1 -> PitchControl/10(P_InitAngle)
  GearboxRatio/1 -> PitchControl/12(GearboxRatio)
  P_StartupSpeed/1 -> PitchControl/13(P_StartUpSpeed)
  P_StartupPitchRate/1 -> PitchControl/14(P_StartupPitchRate)
  SpeedC_2/1 -> PitchControl/15(omega_C)
  DemandedTorque/1 -> PitchControl/16(Demanded_torque)
  Measured_Pitch/1 -> GainScheduler/1(MeasuredPitch), PitchControl/4(MeasuredPitch)
  EventType/1 -> PitchControl/18(Event)
  Clock/1 -> PitchControl/17(Clock)
  EventActionTime/1 -> PitchControl/19(EventTime)
  GainScheduler/1(Kp) -> PitchControl/5(KP)
  GainScheduler/2(Ki) -> PitchControl/6(KI)
  [Notch_beta12wn] -> Notch filter/2(beta12wn)
  GainScheduler/3(Notch_beta12wn) -> [Notch_beta12wn]
  Low-pass filter/1(Output) -> Notch filter/1(u)
  Notch filter/1(Out1) -> Notch filter1/1(u)
  GainScheduler/5(LowPassCutOffFreq) -> [LowPassCutOffFreq]
  [LowPassCutOffFreq] -> Low-pass filter/1(LowPassCutOffFreq)
  GainScheduler/4(Notch2_beta12wn) -> [Notch2_beta12wn]
  [Notch2_beta12wn] -> Notch filter1/2(beta12wn)
  Notch filter1/1(Out1) -> PitchControl/1(GeneratorSpeedError)

== system ClosedLoop_V1/Controller/Shaft Torsion Control ==
  Generator_Speed : Inport
  Gain : Gain  Gain=0
  Generator_Torque : Outport  VectorParamsAs1DForOutWhenUnconnected=off
  wires:
  Generator_Speed/1 -> Gain/1
  Gain/1 -> Generator_Torque/1

== system ClosedLoop_V1/Controller/Sidewards Tower Control ==
  Sidewards_Tower_Accel : Inport
  Gain : Gain  Gain=0
  Generator Torque : Outport  VectorParamsAs1DForOutWhenUnconnected=off
  wires:
  Sidewards_Tower_Accel/1 -> Gain/1
  Gain/1 -> Generator Torque/1

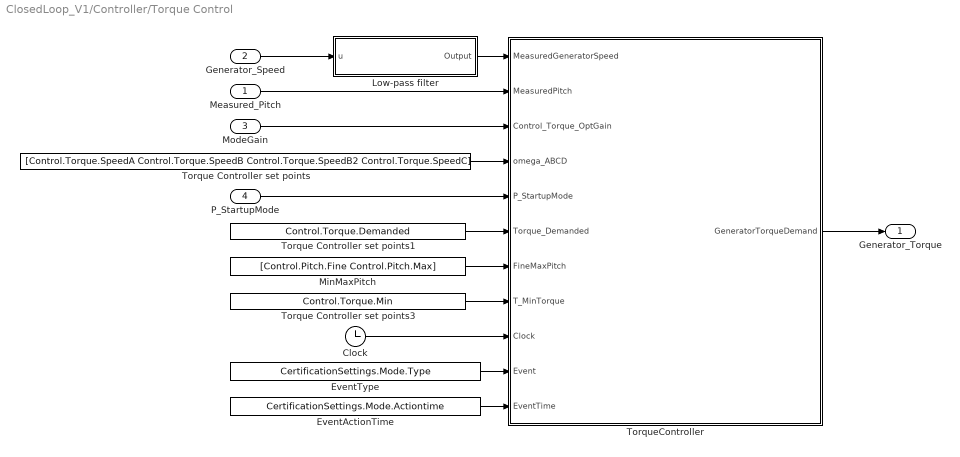
== system ClosedLoop_V1/Controller/Torque Control ==
  Measured_Pitch : Inport
  Generator_Speed : Inport  Port=2
  ModeGain : Inport  Port=3
  P_StartupMode : Inport  Port=4
  Clock : Clock
  EventActionTime : Constant  Value=CertificationSettings.Mode.Actiontime
  EventType : Constant  Value=CertificationSettings.Mode.Type
  Low-pass filter : Subsystem
  MinMaxPitch : Constant  Value=[Control.Pitch.Fine Control.Pitch.Max]
  Torque Controller set points : Constant  Value=[Control.Torque.SpeedA Control.Torque.SpeedB Control.Torque.SpeedB2 Control.Torque.SpeedC]
  Torque Controller set points1 : Constant  Value=Control.Torque.Demanded
  Torque Controller set points3 : Constant  Value=Control.Torque.Min
  TorqueController : MATLAB Function  TreatAsAtomicUnit=on
  Generator_Torque : Outport  VectorParamsAs1DForOutWhenUnconnected=off
  wires:
  Generator_Speed/1 -> Low-pass filter/1(u)
  TorqueController/1(GeneratorTorqueDemand) -> Generator_Torque/1
  Measured_Pitch/1 -> TorqueController/2(MeasuredPitch)
  ModeGain/1 -> TorqueController/3(Control_Torque_OptGain)
  Torque Controller set points/1 -> TorqueController/4(omega_ABCD)
  P_StartupMode/1 -> TorqueController/5(P_StartupMode)
  Low-pass filter/1(Output) -> TorqueController/1(MeasuredGeneratorSpeed)
  Torque Controller set points3/1 -> TorqueController/8(T_MinTorque)
  MinMaxPitch/1 -> TorqueController/7(FineMaxPitch)
  Torque Controller set points1/1 -> TorqueController/6(Torque_Demanded)
  Clock/1 -> TorqueController/9(Clock)
  EventType/1 -> TorqueController/10(Event)
  EventActionTime/1 -> TorqueController/11(EventTime)

== system ClosedLoop_V1/Individual Pitch Controller/Subsystem ==
  M_N2 : Inport
  Derivative : Derivative
  Gain : Gain  Gain=SimConfig.controller.IPC.K_P
  Gain1 : Gain  Gain=SimConfig.controller.IPC.K_D
  Gain3 : Gain  Gain=SimConfig.controller.IPC.K_I
  Integrator : Integrator
  Scope : Scope  NumInputPorts=5
  Scope1 : Scope  NumInputPorts=2
  Scope2 : Scope  NumInputPorts=2
  Scope3 : Scope  NumInputPorts=2
  Sum : Sum  Inputs=+++
  Out1 : Outport  VectorParamsAs1DForOutWhenUnconnected=off
  wires:
  Sum/1 -> Scope/4, Out1/1
  M_N2/1 -> Gain/1, Scope2/2, Gain3/1, Scope/5, Gain1/1  "E"
  Gain/1 -> Scope2/1, Scope/2, Sum/2  "P"
  Integrator/1 -> Scope1/2, Scope/3, Sum/3  "I"
  Derivative/1 -> Sum/1, Scope/1, Scope3/1  "D"
  Gain3/1 -> Integrator/1, Scope1/1
  Gain1/1 -> Derivative/1, Scope3/2

== system ClosedLoop_V1/Individual Pitch Controller/Subsystem1 ==
  M_N3 : Inport
  Derivative : Derivative
  Gain : Gain  Gain=SimConfig.controller.IPC.K_P
  Gain1 : Gain  Gain=SimConfig.controller.IPC.K_D
  Gain3 : Gain  Gain=SimConfig.controller.IPC.K_I
  Integrator : Integrator
  Scope : Scope  NumInputPorts=3
  Scope1 : Scope  NumInputPorts=2
  Scope2 : Scope  NumInputPorts=2
  Scope3 : Scope  NumInputPorts=2
  Sum : Sum  Inputs=+++
  Out1 : Outport  VectorParamsAs1DForOutWhenUnconnected=off
  wires:
  Derivative/1 -> Sum/1, Scope/1, Scope3/1  "D"
  Integrator/1 -> Scope/3, Sum/3, Scope1/2  "I"
  Gain/1 -> Sum/2, Scope/2, Scope2/1  "P"
  M_N3/1 -> Gain1/1, Scope2/2, Gain/1, Gain3/1
  Sum/1 -> Out1/1
  Gain3/1 -> Integrator/1, Scope1/1
  Gain1/1 -> Derivative/1, Scope3/2

== system ClosedLoop_V1/Plot aerodynamic Data/Plot Angle of Attack ==
  OutData : Inport
  Scope1 : Scope  NumInputPorts=9
  Scope10 : Scope  NumInputPorts=3
  Scope12 : Scope  NumInputPorts=3
  Scope16 : Scope  NumInputPorts=3
  extract Angle of Attack : Fcn  Expr=u(strmatch('B1N1Alpha',OutList))
  extract Angle of Attack1 : Fcn  Expr=u(strmatch('B1N2Alpha',OutList))
  extract Angle of Attack2 : Fcn  Expr=u(strmatch('B1N3Alpha',OutList))
  extract Angle of Attack3 : Fcn  Expr=u(strmatch('B1N4Alpha',OutList))
  extract Angle of Attack4 : Fcn  Expr=u(strmatch('B1N5Alpha',OutList))
  extract Angle of Attack5 : Fcn  Expr=u(strmatch('B1N6Alpha',OutList))
  extract Angle of Attack6 : Fcn  Expr=u(strmatch('B1N7Alpha',OutList))
  extract Angle of Attack7 : Fcn  Expr=u(strmatch('B1N8Alpha',OutList))
  extract Angle of Attack8 : Fcn  Expr=u(strmatch('B1N9Alpha',OutList))
  wires:
  OutData/1 -> extract Angle of Attack8/1, extract Angle of Attack7/1, extract Angle of Attack6/1, extract Angle of Attack5/1, extract Angle of Attack4/1, extract Angle of Attack3/1, extract Angle of Attack2/1, extract Angle of Attack1/1, extract Angle of Attack/1
  extract Angle of Attack7/1 -> Scope1/8, Scope16/2  "Angle of Attack (deg)"
  extract Angle of Attack4/1 -> Scope1/5, Scope12/2  "Angle of Attack (deg)"
  extract Angle of Attack8/1 -> Scope1/9, Scope16/3  "Angle of Attack (deg)"
  extract Angle of Attack6/1 -> Scope1/7, Scope16/1  "Angle of Attack (deg)"
  extract Angle of Attack1/1 -> Scope1/2, Scope10/2  "Angle of Attack (deg)"
  extract Angle of Attack3/1 -> Scope1/4, Scope12/1  "Angle of Attack (deg)"
  extract Angle of Attack5/1 -> Scope1/6, Scope12/3  "Angle of Attack (deg)"
  extract Angle of Attack/1 -> Scope1/1, Scope10/1  "Angle of Attack (deg)"
  extract Angle of Attack2/1 -> Scope1/3, Scope10/3  "Angle of Attack (deg)"

== system ClosedLoop_V1/Plot aerodynamic Data/Plot Cd ==
  OutData : Inport
  Scope1 : Scope  NumInputPorts=9
  extract Cd : Fcn  Expr=u(strmatch('B1N1Cd',OutList))
  extract Cd1 : Fcn  Expr=u(strmatch('B1N2Cd',OutList))
  extract Cd2 : Fcn  Expr=u(strmatch('B1N3Cd',OutList))
  extract Cd3 : Fcn  Expr=u(strmatch('B1N4Cd',OutList))
  extract Cd4 : Fcn  Expr=u(strmatch('B1N5Cd',OutList))
  extract Cd5 : Fcn  Expr=u(strmatch('B1N6Cd',OutList))
  extract Cd6 : Fcn  Expr=u(strmatch('B1N7Cd',OutList))
  extract Cd7 : Fcn  Expr=u(strmatch('B1N8Cd',OutList))
  extract Cd8 : Fcn  Expr=u(strmatch('B1N9Cd',OutList))
  wires:
  OutData/1 -> extract Cd4/1, extract Cd5/1, extract Cd6/1, extract Cd8/1, extract Cd7/1, extract Cd3/1, extract Cd2/1, extract Cd1/1, extract Cd/1
  extract Cd/1 -> Scope1/1  "Cd"
  extract Cd1/1 -> Scope1/2  "Cd"
  extract Cd3/1 -> Scope1/4  "Cd"
  extract Cd2/1 -> Scope1/3  "Cd"
  extract Cd4/1 -> Scope1/5  "Cd"
  extract Cd5/1 -> Scope1/6  "Cd"
  extract Cd6/1 -> Scope1/7  "Cd"
  extract Cd7/1 -> Scope1/8  "Cd"
  extract Cd8/1 -> Scope1/9  "Cd"
